simulink model "TDMA"  (R2021a)
settings: Solver=FixedStepDiscrete  StartTime=0.0  StopTime=1e-4  FixedStep=1/(sampling_freq*5)  RelTol=1e-3
undefined symbols (not defined in the file): coeff_t, data_rate, nco_2, nco_costasloopt, nco_t, sample_ratio, sampling_freq
libraries: simulink x64, simulink_extras x14, dspswit3 x14, commrandsrc3 x5
(part 1 of 2)
settings Model: Creator=Administrator  LastModifiedBy=Administrator

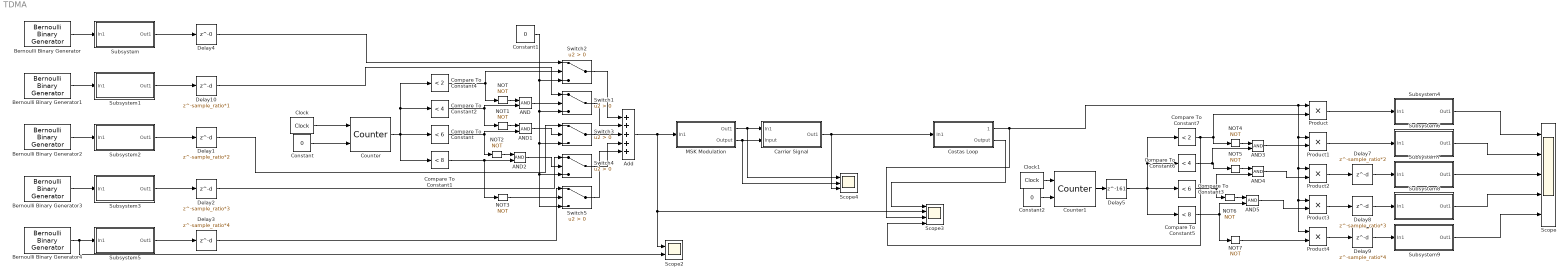
== system TDMA ==
  AND{,1..5} (6 alike) : Logic  IconShape=distinctive  AllPortsSameDT=off  OutDataTypeStr=boolean
  Add : Sum  Inputs=+++++
  Bernoulli Binary Generator{,1..4} (5 alike) : commrandsrc3/Bernoulli Binary Generator  ProbabilityOfZero=0.5  SeedSource=Parameter  Seed=23  SampleTime=1/data_rate  SamplesPerFrame=1  OutputDataType=boolean  SimulateUsing=Interpreted execution
  Carrier Signal : Subsystem
  Clock : simulink_extras/Flip Flops/Clock  period=10/sampling_freq
  Clock1 : simulink_extras/Flip Flops/Clock  period=10/sampling_freq
  Compare To Constant : simulink/Logic and Bit Operations/Compare To Constant  relop=<  const=6  OutDataTypeStr=boolean
  Compare To Constant1 : simulink/Logic and Bit Operations/Compare To Constant  relop=<  const=8  OutDataTypeStr=boolean
  Compare To Constant2 : simulink/Logic and Bit Operations/Compare To Constant  relop=<  const=4  OutDataTypeStr=boolean
  Compare To Constant3 : simulink/Logic and Bit Operations/Compare To Constant  relop=<  const=6  OutDataTypeStr=boolean
  Compare To Constant4 : simulink/Logic and Bit Operations/Compare To Constant  relop=<  const=2  OutDataTypeStr=boolean
  Compare To Constant5 : simulink/Logic and Bit Operations/Compare To Constant  relop=<  const=8  OutDataTypeStr=boolean
  Compare To Constant6 : simulink/Logic and Bit Operations/Compare To Constant  relop=<  const=4  OutDataTypeStr=boolean
  Compare To Constant7 : simulink/Logic and Bit Operations/Compare To Constant  relop=<  const=2  OutDataTypeStr=boolean
  Constant : Constant  Value=0
  Constant1 : Constant  Value=0  SampleTime=25e-9
  Constant2 : Constant  Value=0
  Costas Loop : Subsystem
  Counter : dspswit3/Counter  Direction=Up  CountEvent=Rising edge  CounterSize=User defined  MaxCount=9  InitialCount=0  Output=Count  HitValue=32  ResetInput=on  SamplesPerFrame=1  Ts=1  CntDtype=double  HitDtype=Logical
  Counter1 : dspswit3/Counter  Direction=Up  CountEvent=Rising edge  CounterSize=User defined  MaxCount=9  InitialCount=0  Output=Count  HitValue=32  ResetInput=on  SamplesPerFrame=1  Ts=1  CntDtype=double  HitDtype=Logical
  Delay1 : Delay  DelayLength=sample_ratio*2  SampleTime=1/sampling_freq
  Delay10 : Delay  DelayLength=sample_ratio*1  SampleTime=1/sampling_freq
  Delay2 : Delay  DelayLength=sample_ratio*3  SampleTime=1/sampling_freq
  Delay3 : Delay  DelayLength=sample_ratio*4  SampleTime=1/sampling_freq
  Delay4 : Delay  DelayLength=0  SampleTime=1/sampling_freq
  Delay5 : Delay  DelayLength=161  InitialCondition=0  UseCircularBuffer=on  SampleTime=1/(sampling_freq*5)
  Delay7 : Delay  DelayLength=sample_ratio*2  SampleTime=1/sampling_freq
  Delay8 : Delay  DelayLength=sample_ratio*3  SampleTime=1/sampling_freq
  Delay9 : Delay  DelayLength=sample_ratio*4  SampleTime=1/sampling_freq
  MSK Modulation : Subsystem
  NOT{,1..7} (8 alike) : Logic  Operator=NOT  IconShape=distinctive  AllPortsSameDT=off  OutDataTypeStr=boolean
  Product{,1..4} (5 alike) : Product
  Scope : Scope  NumInputPorts=5
  Scope2 : Scope  NumInputPorts=2
  Scope3 : Scope  NumInputPorts=4
  Scope4 : Scope  NumInputPorts=3
  Subsystem : Subsystem
  Subsystem1 : Subsystem
  Subsystem2 : Subsystem
  Subsystem3 : Subsystem
  Subsystem4 : Subsystem
  Subsystem5 : Subsystem
  Subsystem6 : Subsystem
  Subsystem7 : Subsystem
  Subsystem8 : Subsystem
  Subsystem9 : Subsystem
  Switch{1..5} (5 alike) : Switch  Criteria=u2 > Threshold  OutDataTypeStr=fixdt(1,32,29)  RndMeth=Nearest
  wires:
  Bernoulli Binary Generator/1 -> Subsystem/1(In1)
  Bernoulli Binary Generator1/1 -> Subsystem1/1(In1)
  Bernoulli Binary Generator2/1 -> Subsystem2/1(In1)
  Bernoulli Binary Generator3/1 -> Subsystem3/1(In1)
  Bernoulli Binary Generator4/1 -> Scope2/2, Subsystem5/1(In1)
  MSK Modulation/1(Out1) -> Scope4/1, Carrier Signal/1(In1)
  MSK Modulation/2(Output) -> Scope4/2, Carrier Signal/2(Input)
  Subsystem1/1(Out1) -> Delay10/1
  Subsystem2/1(Out1) -> Delay1/1
  Subsystem3/1(Out1) -> Delay2/1
  Subsystem5/1(Out1) -> Delay3/1
  Switch4/1 -> Add/4
  Switch1/1 -> Add/2
  Counter/1 -> Compare To Constant/1, Compare To Constant1/1, Compare To Constant4/1, Compare To Constant2/1
  Compare To Constant4/1 -> Switch2/2, NOT/1
  Constant1/1 -> Switch4/3, Switch5/3, Switch3/3, Switch1/3, Switch2/3
  Switch2/1 -> Add/1
  Switch3/1 -> Add/3
  Switch5/1 -> Add/5
  Subsystem/1(Out1) -> Delay4/1
  Clock/1 -> Counter/1
  AND/1 -> Switch1/2
  Compare To Constant2/1 -> NOT1/1, AND/2
  NOT/1 -> AND/1
  NOT1/1 -> AND1/1
  Compare To Constant/1 -> AND1/2, NOT2/1
  AND1/1 -> Switch3/2
  NOT2/1 -> AND2/1
  Compare To Constant1/1 -> NOT3/1, AND2/2
  AND2/1 -> Switch4/2
  Constant/1 -> Counter/2
  NOT3/1 -> Switch5/2
  Delay4/1 -> Switch2/1
  Delay10/1 -> Switch1/1
  Delay1/1 -> Switch3/1
  Delay2/1 -> Switch4/1
  Delay3/1 -> Switch5/1
  Constant2/1 -> Counter1/2
  Counter1/1 -> Delay5/1
  Clock1/1 -> Counter1/1
  NOT6/1 -> AND5/1
  NOT5/1 -> AND4/1
  NOT4/1 -> AND3/1
  Compare To Constant5/1 -> NOT7/1, AND5/2
  AND5/1 -> Product3/2
  NOT7/1 -> Product4/2
  Compare To Constant3/1 -> NOT6/1, AND4/2
  Compare To Constant6/1 -> AND3/2, NOT5/1
  Compare To Constant7/1 -> Scope3/4, NOT4/1, Product/2
  AND3/1 -> Product1/2
  AND4/1 -> Product2/2
  Add/1 -> Scope2/1, Scope3/2, MSK Modulation/1(In1)
  Carrier Signal/1(Out1) -> Scope4/3, Costas Loop/1(In1)
  Costas Loop/1(1) -> Scope3/3, Product2/1, Product3/1, Product4/1, Product1/1, Product/1
  Product/1 -> Subsystem4/1(In1)
  Costas Loop/2(Output) -> Scope3/1
  Delay5/1 -> Compare To Constant3/1, Compare To Constant5/1, Compare To Constant7/1, Compare To Constant6/1
  Product2/1 -> Delay7/1
  Product3/1 -> Delay8/1
  Product4/1 -> Delay9/1
  Product1/1 -> Subsystem6/1(In1)
  Delay7/1 -> Subsystem7/1(In1)
  Delay8/1 -> Subsystem8/1(In1)
  Delay9/1 -> Subsystem9/1(In1)
  Subsystem4/1(Out1) -> Scope/1
  Subsystem6/1(Out1) -> Scope/2
  Subsystem7/1(Out1) -> Scope/3
  Subsystem8/1(Out1) -> Scope/4
  Subsystem9/1(Out1) -> Scope/5

== system TDMA/Carrier Signal ==
  In1 : Inport
  Input : Inport  Port=2
  Add : Sum
  Data Type Conversion1 : DataTypeConversion  OutMin=[-1]  OutMax=[1]  OutDataTypeStr=fixdt(1,8)
  Data Type Conversion2 : DataTypeConversion  OutMin=[-1]  OutMax=[1]  OutDataTypeStr=fixdt(1,8)
  Data Type Conversion36 : DataTypeConversion  OutMin=[-2]  OutMax=[2]  OutDataTypeStr=fixdt(1,16)
  NCO : Subsystem
  Product2 : Product
  Product3 : Product
  Out1 : Outport
  wires:
  In1/1 -> Product3/2
  Data Type Conversion2/1 -> Product3/1
  NCO/1(Out2) -> Data Type Conversion2/1
  Product2/1 -> Add/2
  Add/1 -> Data Type Conversion36/1
  Product3/1 -> Add/1
  NCO/2(Out1) -> Data Type Conversion1/1
  Input/1 -> Product2/1
  Data Type Conversion1/1 -> Product2/2
  Data Type Conversion36/1 -> Out1/1

== system TDMA/Costas Loop ==
  In1 : Inport
  Compare To Constant4 : simulink/Logic and Bit Operations/Compare To Constant  relop=>  const=0  OutDataTypeStr=boolean
  Data Type Conversion{32..35,37..38} (6 alike) : DataTypeConversion  OutMin=[-2]  OutMax=[2]  OutDataTypeStr=fixdt(1,16)
  Filter1 : Subsystem  Tag=FilterWizardSubSystem
      settings: ErrorFcn=dspFilterRealizedInBasicElemsAlgLoopErrFcnCallback
  Filter2 : Subsystem  Tag=FilterWizardSubSystem
      settings: ErrorFcn=dspFilterRealizedInBasicElemsAlgLoopErrFcnCallback
  Filter3 : Subsystem  Tag=FilterWizardSubSystem
      settings: ErrorFcn=dspFilterRealizedInBasicElemsAlgLoopErrFcnCallback
  Gain : Gain  Gain=1/100
  NCO1 : Subsystem
  Product10 : Product
  Product11 : Product
  Product9 : Product
  Scope : Scope  NumInputPorts=2
  1 : Outport
  Output : Outport  Port=2
  wires:
  Data Type Conversion38/1 -> NCO1/1(In1)
  Data Type Conversion33/1 -> Product11/2
  Filter3/1(Output) -> Compare To Constant4/1, Product10/2, Output/1, Scope/1
  Filter1/1(Output) -> Product10/1, Scope/2
  Data Type Conversion32/1 -> Filter3/1(Input)
  Data Type Conversion34/1 -> Product9/1
  Filter2/1(Output) -> Gain/1
  NCO1/1(Out1) -> Product9/2
  Data Type Conversion37/1 -> Filter2/1(Input)
  In1/1 -> Data Type Conversion34/1, Data Type Conversion33/1
  Gain/1 -> Data Type Conversion38/1
  Product10/1 -> Data Type Conversion37/1
  Product11/1 -> Data Type Conversion32/1
  Data Type Conversion35/1 -> Filter1/1(Input)
  Compare To Constant4/1 -> 1/1
  Product9/1 -> Data Type Conversion35/1
  NCO1/2(sin(2*pi*u)) -> Product11/1

== system TDMA/MSK Modulation ==
  In1 : Inport
  Add1 : Sum
  Add2 : Sum
  Constant : Constant  Value=-1
  Constant1 : Constant  Value=2
  Constant2 : Constant  Value=-1
  Constant3 : Constant  Value=2
  Data Type Conversion : DataTypeConversion  OutDataTypeStr=boolean
  Data Type Conversion{3..6} (4 alike) : DataTypeConversion  OutMin=[-1]  OutMax=[1]  OutDataTypeStr=fixdt(1,8)
  Delay : Delay  DelayLength=sample_ratio  SampleTime=1/(sampling_freq*5)
  Delay1 : Delay  DelayLength=sample_ratio  SampleTime=1/(sampling_freq*5)
  NCO2 : Subsystem
  Product{,1,4..5} (4 alike) : Product
  clock : DiscretePulseGenerator  PulseType=Time based  Period=2/(sampling_freq*5)  PulseWidth=50
  rate transition1 : Subsystem
  rate transition3 : Subsystem
  Out1 : Outport
  Output : Outport  Port=2
  wires:
  NCO2/2(Out1) -> Data Type Conversion3/1
  Delay/1 -> rate transition1/1(In1)
  Delay1/1 -> Product4/2
  rate transition1/1(Out1) -> Product5/2
  rate transition3/1(Out1) -> Delay1/1
  NCO2/1(Out2) -> Data Type Conversion6/1
  Data Type Conversion6/1 -> Product1/1
  Add2/1 -> Data Type Conversion4/1
  Data Type Conversion4/1 -> Product/1
  Data Type Conversion3/1 -> Product/2
  Constant1/1 -> Product4/1
  Data Type Conversion5/1 -> Product1/2
  Add1/1 -> Data Type Conversion5/1
  Product5/1 -> Add2/2
  Data Type Conversion/1 -> rate transition3/1(In1), Delay/1
  clock/1 -> rate transition1/2(In2), rate transition3/2(In2)
  Constant2/1 -> Add2/1
  Constant/1 -> Add1/1
  Constant3/1 -> Product5/1
  Product4/1 -> Add1/2
  Product1/1 -> Out1/1
  Product/1 -> Output/1
  In1/1 -> Data Type Conversion/1

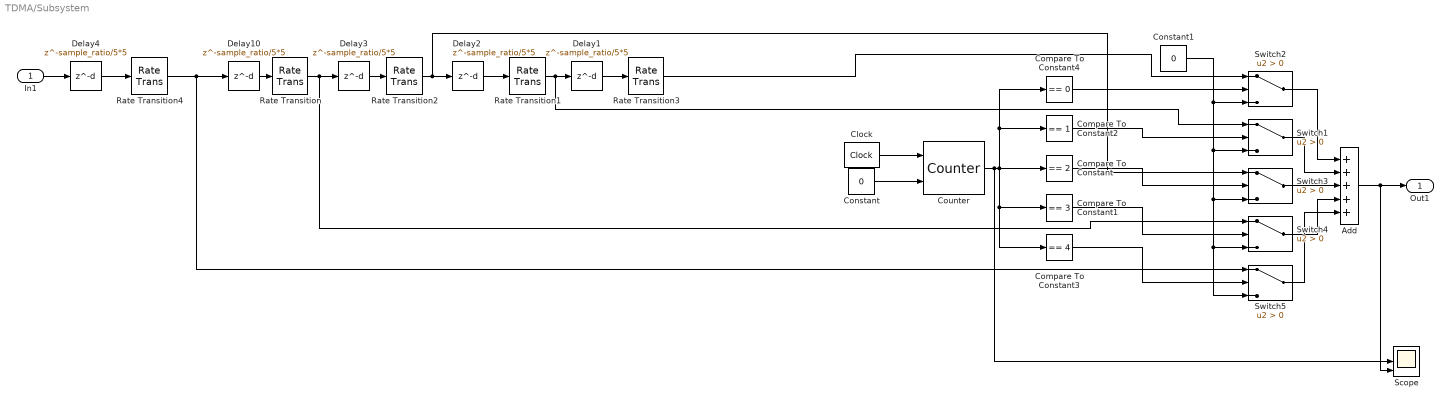
== system TDMA/Subsystem ==
  In1 : Inport
  Add : Sum  Inputs=+++++
  Clock : simulink_extras/Flip Flops/Clock  period=4/sampling_freq
  Compare To Constant : simulink/Logic and Bit Operations/Compare To Constant  relop===  const=2  OutDataTypeStr=boolean
  Compare To Constant1 : simulink/Logic and Bit Operations/Compare To Constant  relop===  const=3  OutDataTypeStr=boolean
  Compare To Constant2 : simulink/Logic and Bit Operations/Compare To Constant  relop===  const=1  OutDataTypeStr=boolean
  Compare To Constant3 : simulink/Logic and Bit Operations/Compare To Constant  relop===  const=4  OutDataTypeStr=boolean
  Compare To Constant4 : simulink/Logic and Bit Operations/Compare To Constant  relop===  const=0  OutDataTypeStr=boolean
  Constant : Constant  Value=0
  Constant1 : Constant  Value=0  SampleTime=25e-9
  Counter : dspswit3/Counter  Direction=Up  CountEvent=Rising edge  CounterSize=User defined  MaxCount=4  InitialCount=0  Output=Count  HitValue=32  ResetInput=on  SamplesPerFrame=1  Ts=1  CntDtype=double  HitDtype=Logical
  Delay{1..4,10} (5 alike) : Delay  DelayLength=sample_ratio/5*5  SampleTime=1/sampling_freq
  Rate Transition{,1..4} (5 alike) : RateTransition  OutPortSampleTime=1/data_rate
  Scope : Scope  NumInputPorts=3
  Switch{1..5} (5 alike) : Switch  Criteria=u2 > Threshold  OutDataTypeStr=fixdt(1,32,29)  RndMeth=Nearest
  Out1 : Outport
  wires:
  Rate Transition1/1 -> Switch1/1, Delay1/1
  Switch2/1 -> Add/1
  Counter/1 -> Scope/2, Compare To Constant/1, Compare To Constant3/1, Compare To Constant1/1, Compare To Constant4/1, Compare To Constant2/1
  Delay2/1 -> Rate Transition1/1
  Add/1 -> Scope/3, Out1/1
  Constant/1 -> Counter/2
  Switch3/1 -> Add/3
  Constant1/1 -> Switch4/3, Switch5/3, Switch3/3, Switch1/3, Switch2/3
  Switch5/1 -> Add/5
  Rate Transition/1 -> Switch4/1, Delay3/1
  Switch4/1 -> Add/4
  Delay3/1 -> Rate Transition2/1
  Compare To Constant2/1 -> Switch1/2
  Compare To Constant3/1 -> Switch5/2
  Compare To Constant/1 -> Switch3/2
  Switch1/1 -> Add/2
  Clock/1 -> Counter/1
  Compare To Constant1/1 -> Switch4/2
  Delay1/1 -> Rate Transition3/1
  Rate Transition2/1 -> Switch3/1, Delay2/1
  Compare To Constant4/1 -> Switch2/2
  Delay10/1 -> Rate Transition/1
  In1/1 -> Delay4/1
  Rate Transition3/1 -> Switch2/1
  Rate Transition4/1 -> Switch5/1, Delay10/1
  Delay4/1 -> Rate Transition4/1

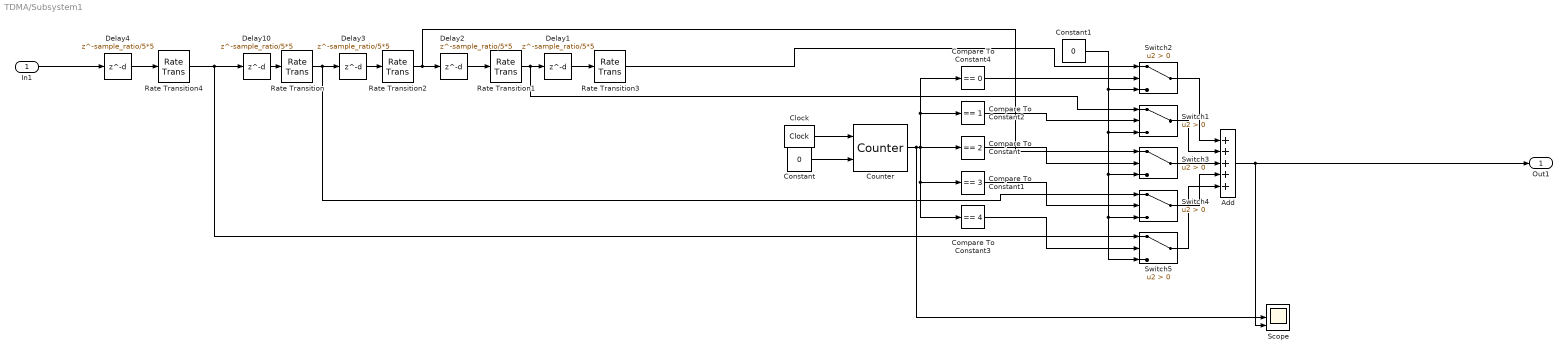
== system TDMA/Subsystem1 ==
  In1 : Inport
  Add : Sum  Inputs=+++++
  Clock : simulink_extras/Flip Flops/Clock  period=4/sampling_freq
  Compare To Constant : simulink/Logic and Bit Operations/Compare To Constant  relop===  const=2  OutDataTypeStr=boolean
  Compare To Constant1 : simulink/Logic and Bit Operations/Compare To Constant  relop===  const=3  OutDataTypeStr=boolean
  Compare To Constant2 : simulink/Logic and Bit Operations/Compare To Constant  relop===  const=1  OutDataTypeStr=boolean
  Compare To Constant3 : simulink/Logic and Bit Operations/Compare To Constant  relop===  const=4  OutDataTypeStr=boolean
  Compare To Constant4 : simulink/Logic and Bit Operations/Compare To Constant  relop===  const=0  OutDataTypeStr=boolean
  Constant : Constant  Value=0
  Constant1 : Constant  Value=0  SampleTime=25e-9
  Counter : dspswit3/Counter  Direction=Up  CountEvent=Rising edge  CounterSize=User defined  MaxCount=4  InitialCount=0  Output=Count  HitValue=32  ResetInput=on  SamplesPerFrame=1  Ts=1  CntDtype=double  HitDtype=Logical
  Delay{1..4,10} (5 alike) : Delay  DelayLength=sample_ratio/5*5  SampleTime=1/sampling_freq
  Rate Transition{,1..4} (5 alike) : RateTransition  OutPortSampleTime=1/data_rate
  Scope : Scope  NumInputPorts=3
  Switch{1..5} (5 alike) : Switch  Criteria=u2 > Threshold  OutDataTypeStr=fixdt(1,32,29)  RndMeth=Nearest
  Out1 : Outport
  wires:
  Rate Transition1/1 -> Switch1/1, Delay1/1
  Switch2/1 -> Add/1
  Counter/1 -> Scope/2, Compare To Constant/1, Compare To Constant3/1, Compare To Constant1/1, Compare To Constant4/1, Compare To Constant2/1
  Delay2/1 -> Rate Transition1/1
  Add/1 -> Scope/3, Out1/1
  Constant/1 -> Counter/2
  Switch3/1 -> Add/3
  Constant1/1 -> Switch4/3, Switch5/3, Switch3/3, Switch1/3, Switch2/3
  Switch5/1 -> Add/5
  Rate Transition/1 -> Switch4/1, Delay3/1
  Switch4/1 -> Add/4
  Delay3/1 -> Rate Transition2/1
  Compare To Constant2/1 -> Switch1/2
  Compare To Constant3/1 -> Switch5/2
  Compare To Constant/1 -> Switch3/2
  Switch1/1 -> Add/2
  Clock/1 -> Counter/1
  Compare To Constant1/1 -> Switch4/2
  Delay1/1 -> Rate Transition3/1
  Rate Transition2/1 -> Switch3/1, Delay2/1
  Compare To Constant4/1 -> Switch2/2
  Delay10/1 -> Rate Transition/1
  In1/1 -> Delay4/1
  Rate Transition3/1 -> Switch2/1
  Rate Transition4/1 -> Switch5/1, Delay10/1
  Delay4/1 -> Rate Transition4/1

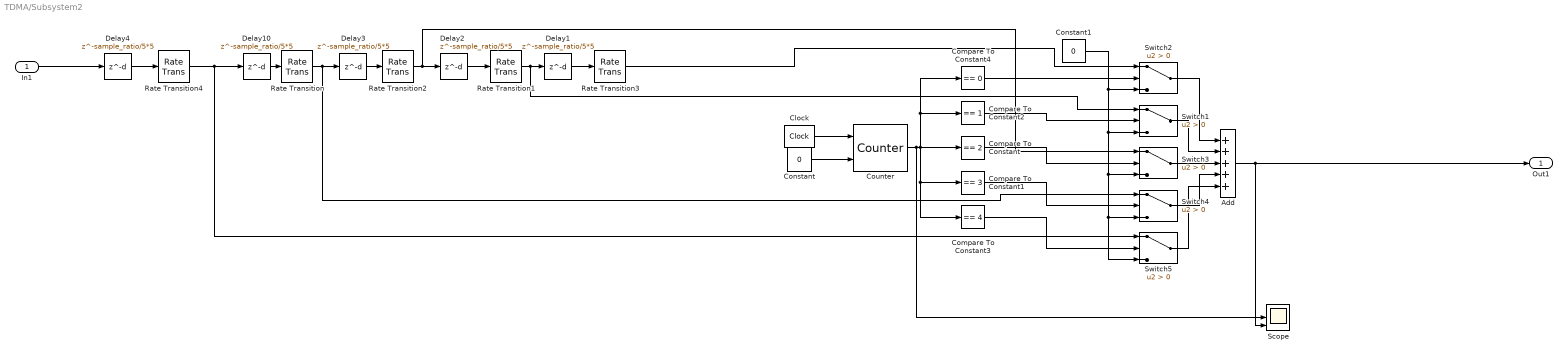
== system TDMA/Subsystem2 ==
  In1 : Inport
  Add : Sum  Inputs=+++++
  Clock : simulink_extras/Flip Flops/Clock  period=4/sampling_freq
  Compare To Constant : simulink/Logic and Bit Operations/Compare To Constant  relop===  const=2  OutDataTypeStr=boolean
  Compare To Constant1 : simulink/Logic and Bit Operations/Compare To Constant  relop===  const=3  OutDataTypeStr=boolean
  Compare To Constant2 : simulink/Logic and Bit Operations/Compare To Constant  relop===  const=1  OutDataTypeStr=boolean
  Compare To Constant3 : simulink/Logic and Bit Operations/Compare To Constant  relop===  const=4  OutDataTypeStr=boolean
  Compare To Constant4 : simulink/Logic and Bit Operations/Compare To Constant  relop===  const=0  OutDataTypeStr=boolean
  Constant : Constant  Value=0
  Constant1 : Constant  Value=0  SampleTime=25e-9
  Counter : dspswit3/Counter  Direction=Up  CountEvent=Rising edge  CounterSize=User defined  MaxCount=4  InitialCount=0  Output=Count  HitValue=32  ResetInput=on  SamplesPerFrame=1  Ts=1  CntDtype=double  HitDtype=Logical
  Delay{1..4,10} (5 alike) : Delay  DelayLength=sample_ratio/5*5  SampleTime=1/sampling_freq
  Rate Transition{,1..4} (5 alike) : RateTransition  OutPortSampleTime=1/data_rate
  Scope : Scope  NumInputPorts=3
  Switch{1..5} (5 alike) : Switch  Criteria=u2 > Threshold  OutDataTypeStr=fixdt(1,32,29)  RndMeth=Nearest
  Out1 : Outport
  wires:
  Rate Transition1/1 -> Switch1/1, Delay1/1
  Switch2/1 -> Add/1
  Counter/1 -> Scope/2, Compare To Constant/1, Compare To Constant3/1, Compare To Constant1/1, Compare To Constant4/1, Compare To Constant2/1
  Delay2/1 -> Rate Transition1/1
  Add/1 -> Scope/3, Out1/1
  Constant/1 -> Counter/2
  Switch3/1 -> Add/3
  Constant1/1 -> Switch4/3, Switch5/3, Switch3/3, Switch1/3, Switch2/3
  Switch5/1 -> Add/5
  Rate Transition/1 -> Switch4/1, Delay3/1
  Switch4/1 -> Add/4
  Delay3/1 -> Rate Transition2/1
  Compare To Constant2/1 -> Switch1/2
  Compare To Constant3/1 -> Switch5/2
  Compare To Constant/1 -> Switch3/2
  Switch1/1 -> Add/2
  Clock/1 -> Counter/1
  Compare To Constant1/1 -> Switch4/2
  Delay1/1 -> Rate Transition3/1
  Rate Transition2/1 -> Switch3/1, Delay2/1
  Compare To Constant4/1 -> Switch2/2
  Delay10/1 -> Rate Transition/1
  In1/1 -> Delay4/1
  Rate Transition3/1 -> Switch2/1
  Rate Transition4/1 -> Switch5/1, Delay10/1
  Delay4/1 -> Rate Transition4/1

== system TDMA/Subsystem3 ==
  In1 : Inport
  Add : Sum  Inputs=+++++
  Clock : simulink_extras/Flip Flops/Clock  period=4/sampling_freq
  Compare To Constant : simulink/Logic and Bit Operations/Compare To Constant  relop===  const=2  OutDataTypeStr=boolean
  Compare To Constant1 : simulink/Logic and Bit Operations/Compare To Constant  relop===  const=3  OutDataTypeStr=boolean
  Compare To Constant2 : simulink/Logic and Bit Operations/Compare To Constant  relop===  const=1  OutDataTypeStr=boolean
  Compare To Constant3 : simulink/Logic and Bit Operations/Compare To Constant  relop===  const=4  OutDataTypeStr=boolean
  Compare To Constant4 : simulink/Logic and Bit Operations/Compare To Constant  relop===  const=0  OutDataTypeStr=boolean
  Constant : Constant  Value=0
  Constant1 : Constant  Value=0  SampleTime=25e-9
  Counter : dspswit3/Counter  Direction=Up  CountEvent=Rising edge  CounterSize=User defined  MaxCount=4  InitialCount=0  Output=Count  HitValue=32  ResetInput=on  SamplesPerFrame=1  Ts=1  CntDtype=double  HitDtype=Logical
  Delay{1..4,10} (5 alike) : Delay  DelayLength=sample_ratio/5*5  SampleTime=1/sampling_freq
  Rate Transition{,1..4} (5 alike) : RateTransition  OutPortSampleTime=1/data_rate
  Scope : Scope  NumInputPorts=3
  Switch{1..5} (5 alike) : Switch  Criteria=u2 > Threshold  OutDataTypeStr=fixdt(1,32,29)  RndMeth=Nearest
  Out1 : Outport
  wires:
  Rate Transition1/1 -> Switch1/1, Delay1/1
  Switch2/1 -> Add/1
  Counter/1 -> Scope/2, Compare To Constant/1, Compare To Constant3/1, Compare To Constant1/1, Compare To Constant4/1, Compare To Constant2/1
  Delay2/1 -> Rate Transition1/1
  Add/1 -> Scope/3, Out1/1
  Constant/1 -> Counter/2
  Switch3/1 -> Add/3
  Constant1/1 -> Switch4/3, Switch5/3, Switch3/3, Switch1/3, Switch2/3
  Switch5/1 -> Add/5
  Rate Transition/1 -> Switch4/1, Delay3/1
  Switch4/1 -> Add/4
  Delay3/1 -> Rate Transition2/1
  Compare To Constant2/1 -> Switch1/2
  Compare To Constant3/1 -> Switch5/2
  Compare To Constant/1 -> Switch3/2
  Switch1/1 -> Add/2
  Clock/1 -> Counter/1
  Compare To Constant1/1 -> Switch4/2
  Delay1/1 -> Rate Transition3/1
  Rate Transition2/1 -> Switch3/1, Delay2/1
  Compare To Constant4/1 -> Switch2/2
  Delay10/1 -> Rate Transition/1
  In1/1 -> Delay4/1
  Rate Transition3/1 -> Switch2/1
  Rate Transition4/1 -> Switch5/1, Delay10/1
  Delay4/1 -> Rate Transition4/1

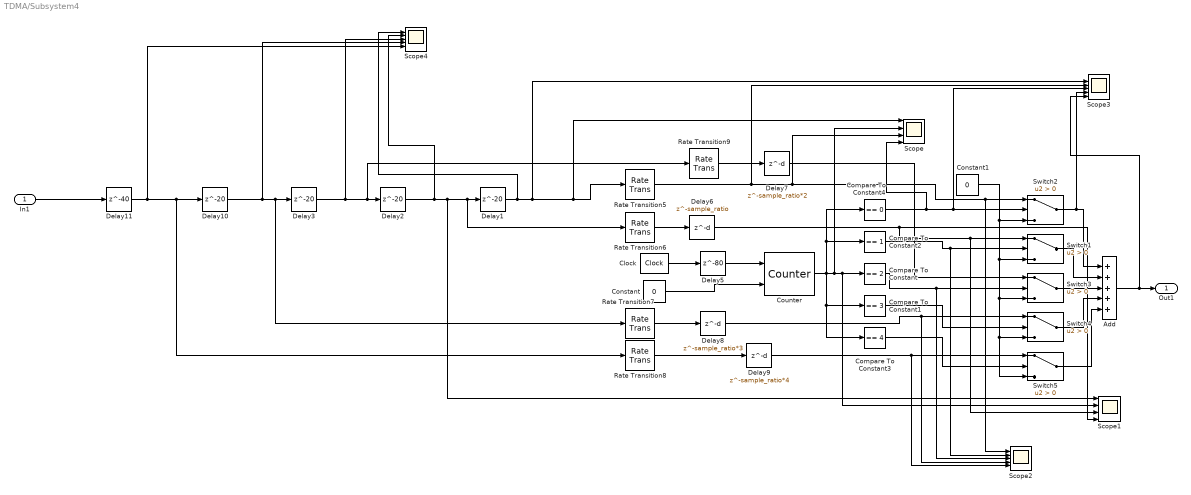
== system TDMA/Subsystem4 ==
  In1 : Inport
  Add : Sum  Inputs=+++++
  Clock : simulink_extras/Flip Flops/Clock  period=5*4/(sampling_freq)
  Compare To Constant : simulink/Logic and Bit Operations/Compare To Constant  relop===  const=2  OutDataTypeStr=boolean
  Compare To Constant1 : simulink/Logic and Bit Operations/Compare To Constant  relop===  const=3  OutDataTypeStr=boolean
  Compare To Constant2 : simulink/Logic and Bit Operations/Compare To Constant  relop===  const=1  OutDataTypeStr=boolean
  Compare To Constant3 : simulink/Logic and Bit Operations/Compare To Constant  relop===  const=4  OutDataTypeStr=boolean
  Compare To Constant4 : simulink/Logic and Bit Operations/Compare To Constant  relop===  const=0  OutDataTypeStr=boolean
  Constant : Constant  Value=0
  Constant1 : Constant  Value=0  SampleTime=25e-9
  Counter : dspswit3/Counter  Direction=Up  CountEvent=Rising edge  CounterSize=User defined  MaxCount=4  InitialCount=0  Output=Count  HitValue=32  ResetInput=on  SamplesPerFrame=1  Ts=1  CntDtype=double  HitDtype=Logical
  Delay{1..3,10} (4 alike) : Delay  DelayLength=20  SampleTime=1/(sampling_freq*5)
  Delay11 : Delay  DelayLength=40  SampleTime=1/(sampling_freq*5)
  Delay5 : Delay  DelayLength=80  SampleTime=1/(sampling_freq)
  Delay6 : Delay  DelayLength=sample_ratio  SampleTime=1/(sampling_freq)
  Delay7 : Delay  DelayLength=sample_ratio*2  SampleTime=1/(sampling_freq)
  Delay8 : Delay  DelayLength=sample_ratio*3  SampleTime=1/(sampling_freq)
  Delay9 : Delay  DelayLength=sample_ratio*4  SampleTime=1/(sampling_freq)
  Rate Transition{5..9} (5 alike) : RateTransition  OutPortSampleTime=1/(data_rate)
  Scope : Scope  NumInputPorts=4
  Scope1 : Scope  NumInputPorts=4
  Scope2 : Scope  NumInputPorts=5
  Scope3 : Scope  NumInputPorts=6
  Scope4 : Scope  NumInputPorts=5
  Switch{1..5} (5 alike) : Switch  Criteria=u2 > Threshold  OutDataTypeStr=fixdt(1,32,29)  RndMeth=Nearest
  Out1 : Outport
  wires:
  Switch2/1 -> Scope3/5, Add/1
  Counter/1 -> Scope/2, Scope1/2, Compare To Constant/1, Compare To Constant3/1, Compare To Constant1/1, Compare To Constant4/1, Compare To Constant2/1
  Add/1 -> Scope3/6, Out1/1
  Constant/1 -> Counter/2
  Switch3/1 -> Add/3
  Constant1/1 -> Switch4/3, Switch5/3, Switch3/3, Switch1/3, Switch2/3
  Switch5/1 -> Add/5
  Switch4/1 -> Add/4
  Compare To Constant2/1 -> Scope2/2, Switch1/2
  Compare To Constant3/1 -> Switch5/2
  Compare To Constant/1 -> Scope2/3, Switch3/2
  Switch1/1 -> Add/2
  Compare To Constant1/1 -> Switch4/2
  Compare To Constant4/1 -> Scope/4, Scope3/4, Switch2/2
  Delay1/1 -> Scope4/1, Scope3/2, Scope/1, Rate Transition5/1
  Rate Transition6/1 -> Delay6/1
  Rate Transition7/1 -> Delay8/1
  Rate Transition8/1 -> Delay9/1
  Rate Transition9/1 -> Delay7/1
  Clock/1 -> Delay5/1
  Delay5/1 -> Counter/1
  Delay2/1 -> Scope4/2, Scope1/1, Rate Transition6/1, Delay1/1
  Delay3/1 -> Scope4/3, Rate Transition9/1, Delay2/1
  Delay10/1 -> Scope4/4, Rate Transition7/1, Delay3/1
  Delay6/1 -> Scope1/4, Scope1/3, Switch1/1
  Delay7/1 -> Switch3/1
  Delay8/1 -> Scope2/4, Switch4/1
  Delay9/1 -> Scope2/5, Switch5/1
  Rate Transition5/1 -> Scope3/3, Scope2/1, Switch2/1, Scope/3
  In1/1 -> Delay11/1
  Delay11/1 -> Scope4/5, Rate Transition8/1, Delay10/1

== system TDMA/Subsystem5 ==
  In1 : Inport
  Add : Sum  Inputs=+++++
  Clock : simulink_extras/Flip Flops/Clock  period=4/sampling_freq
  Compare To Constant : simulink/Logic and Bit Operations/Compare To Constant  relop===  const=2  OutDataTypeStr=boolean
  Compare To Constant1 : simulink/Logic and Bit Operations/Compare To Constant  relop===  const=3  OutDataTypeStr=boolean
  Compare To Constant2 : simulink/Logic and Bit Operations/Compare To Constant  relop===  const=1  OutDataTypeStr=boolean
  Compare To Constant3 : simulink/Logic and Bit Operations/Compare To Constant  relop===  const=4  OutDataTypeStr=boolean
  Compare To Constant4 : simulink/Logic and Bit Operations/Compare To Constant  relop===  const=0  OutDataTypeStr=boolean
  Constant : Constant  Value=0
  Constant1 : Constant  Value=0  SampleTime=25e-9
  Counter : dspswit3/Counter  Direction=Up  CountEvent=Rising edge  CounterSize=User defined  MaxCount=4  InitialCount=0  Output=Count  HitValue=32  ResetInput=on  SamplesPerFrame=1  Ts=1  CntDtype=double  HitDtype=Logical
  Delay{1..4,10} (5 alike) : Delay  DelayLength=sample_ratio/5*5  SampleTime=1/sampling_freq
  Rate Transition{,1..4} (5 alike) : RateTransition  OutPortSampleTime=1/data_rate
  Scope : Scope  NumInputPorts=3
  Switch{1..5} (5 alike) : Switch  Criteria=u2 > Threshold  OutDataTypeStr=fixdt(1,32,29)  RndMeth=Nearest
  Out1 : Outport
  wires:
  Rate Transition1/1 -> Switch1/1, Delay1/1
  Switch2/1 -> Add/1
  Counter/1 -> Scope/2, Compare To Constant/1, Compare To Constant3/1, Compare To Constant1/1, Compare To Constant4/1, Compare To Constant2/1
  Delay2/1 -> Rate Transition1/1
  Add/1 -> Scope/3, Out1/1
  Constant/1 -> Counter/2
  Switch3/1 -> Add/3
  Constant1/1 -> Switch4/3, Switch5/3, Switch3/3, Switch1/3, Switch2/3
  Switch5/1 -> Add/5
  Rate Transition/1 -> Switch4/1, Delay3/1
  Switch4/1 -> Add/4
  Delay3/1 -> Rate Transition2/1
  Compare To Constant2/1 -> Switch1/2
  Compare To Constant3/1 -> Switch5/2
  Compare To Constant/1 -> Switch3/2
  Switch1/1 -> Add/2
  Clock/1 -> Counter/1
  Compare To Constant1/1 -> Switch4/2
  Delay1/1 -> Rate Transition3/1
  Rate Transition2/1 -> Switch3/1, Delay2/1
  Compare To Constant4/1 -> Switch2/2
  Delay10/1 -> Rate Transition/1
  In1/1 -> Delay4/1
  Rate Transition3/1 -> Switch2/1
  Rate Transition4/1 -> Switch5/1, Delay10/1
  Delay4/1 -> Rate Transition4/1

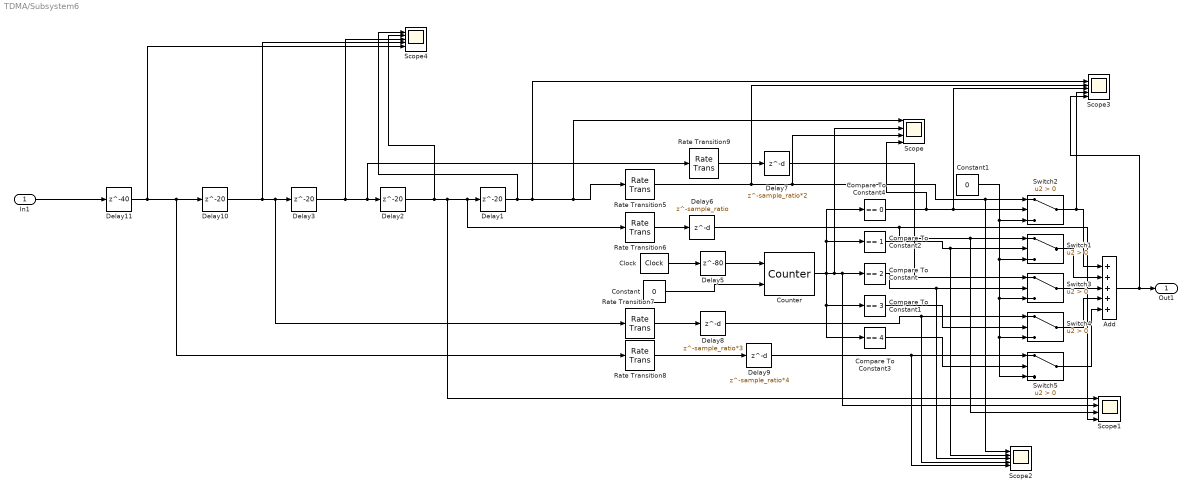
== system TDMA/Subsystem6 ==
  In1 : Inport
  Add : Sum  Inputs=+++++
  Clock : simulink_extras/Flip Flops/Clock  period=5*4/(sampling_freq)
  Compare To Constant : simulink/Logic and Bit Operations/Compare To Constant  relop===  const=2  OutDataTypeStr=boolean
  Compare To Constant1 : simulink/Logic and Bit Operations/Compare To Constant  relop===  const=3  OutDataTypeStr=boolean
  Compare To Constant2 : simulink/Logic and Bit Operations/Compare To Constant  relop===  const=1  OutDataTypeStr=boolean
  Compare To Constant3 : simulink/Logic and Bit Operations/Compare To Constant  relop===  const=4  OutDataTypeStr=boolean
  Compare To Constant4 : simulink/Logic and Bit Operations/Compare To Constant  relop===  const=0  OutDataTypeStr=boolean
  Constant : Constant  Value=0
  Constant1 : Constant  Value=0  SampleTime=25e-9
  Counter : dspswit3/Counter  Direction=Up  CountEvent=Rising edge  CounterSize=User defined  MaxCount=4  InitialCount=0  Output=Count  HitValue=32  ResetInput=on  SamplesPerFrame=1  Ts=1  CntDtype=double  HitDtype=Logical
  Delay{1..3,10} (4 alike) : Delay  DelayLength=20  SampleTime=1/(sampling_freq*5)
  Delay11 : Delay  DelayLength=40  SampleTime=1/(sampling_freq*5)
  Delay5 : Delay  DelayLength=80  SampleTime=1/(sampling_freq)
  Delay6 : Delay  DelayLength=sample_ratio  SampleTime=1/(sampling_freq)
  Delay7 : Delay  DelayLength=sample_ratio*2  SampleTime=1/(sampling_freq)
  Delay8 : Delay  DelayLength=sample_ratio*3  SampleTime=1/(sampling_freq)
  Delay9 : Delay  DelayLength=sample_ratio*4  SampleTime=1/(sampling_freq)
  Rate Transition{5..9} (5 alike) : RateTransition  OutPortSampleTime=1/(data_rate)
  Scope : Scope  NumInputPorts=4
  Scope1 : Scope  NumInputPorts=4
  Scope2 : Scope  NumInputPorts=5
  Scope3 : Scope  NumInputPorts=6
  Scope4 : Scope  NumInputPorts=5
  Switch{1..5} (5 alike) : Switch  Criteria=u2 > Threshold  OutDataTypeStr=fixdt(1,32,29)  RndMeth=Nearest
  Out1 : Outport
  wires:
  Switch2/1 -> Scope3/5, Add/1
  Counter/1 -> Scope/2, Scope1/2, Compare To Constant/1, Compare To Constant3/1, Compare To Constant1/1, Compare To Constant4/1, Compare To Constant2/1
  Add/1 -> Scope3/6, Out1/1
  Constant/1 -> Counter/2
  Switch3/1 -> Add/3
  Constant1/1 -> Switch4/3, Switch5/3, Switch3/3, Switch1/3, Switch2/3
  Switch5/1 -> Add/5
  Switch4/1 -> Add/4
  Compare To Constant2/1 -> Scope2/2, Switch1/2
  Compare To Constant3/1 -> Switch5/2
  Compare To Constant/1 -> Scope2/3, Switch3/2
  Switch1/1 -> Add/2
  Compare To Constant1/1 -> Switch4/2
  Compare To Constant4/1 -> Scope/4, Scope3/4, Switch2/2
  Delay1/1 -> Scope4/1, Scope3/2, Scope/1, Rate Transition5/1
  Rate Transition6/1 -> Delay6/1
  Rate Transition7/1 -> Delay8/1
  Rate Transition8/1 -> Delay9/1
  Rate Transition9/1 -> Delay7/1
  Clock/1 -> Delay5/1
  Delay5/1 -> Counter/1
  Delay2/1 -> Scope4/2, Scope1/1, Rate Transition6/1, Delay1/1
  Delay3/1 -> Scope4/3, Rate Transition9/1, Delay2/1
  Delay10/1 -> Scope4/4, Rate Transition7/1, Delay3/1
  Delay6/1 -> Scope1/4, Scope1/3, Switch1/1
  Delay7/1 -> Switch3/1
  Delay8/1 -> Scope2/4, Switch4/1
  Delay9/1 -> Scope2/5, Switch5/1
  Rate Transition5/1 -> Scope3/3, Scope2/1, Switch2/1, Scope/3
  In1/1 -> Delay11/1
  Delay11/1 -> Scope4/5, Rate Transition8/1, Delay10/1

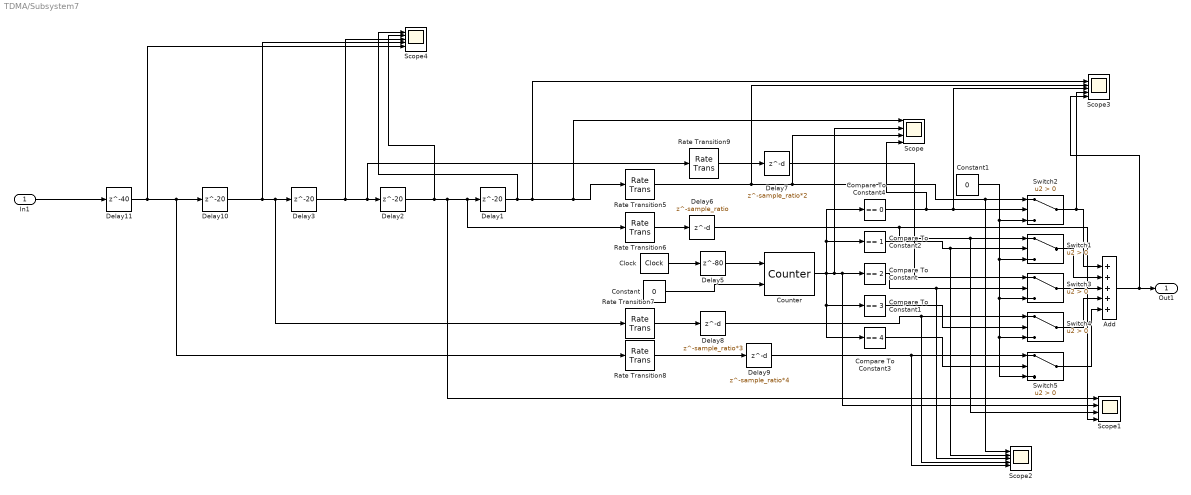
== system TDMA/Subsystem7 ==
  In1 : Inport
  Add : Sum  Inputs=+++++
  Clock : simulink_extras/Flip Flops/Clock  period=5*4/(sampling_freq)
  Compare To Constant : simulink/Logic and Bit Operations/Compare To Constant  relop===  const=2  OutDataTypeStr=boolean
  Compare To Constant1 : simulink/Logic and Bit Operations/Compare To Constant  relop===  const=3  OutDataTypeStr=boolean
  Compare To Constant2 : simulink/Logic and Bit Operations/Compare To Constant  relop===  const=1  OutDataTypeStr=boolean
  Compare To Constant3 : simulink/Logic and Bit Operations/Compare To Constant  relop===  const=4  OutDataTypeStr=boolean
  Compare To Constant4 : simulink/Logic and Bit Operations/Compare To Constant  relop===  const=0  OutDataTypeStr=boolean
  Constant : Constant  Value=0
  Constant1 : Constant  Value=0  SampleTime=25e-9
  Counter : dspswit3/Counter  Direction=Up  CountEvent=Rising edge  CounterSize=User defined  MaxCount=4  InitialCount=0  Output=Count  HitValue=32  ResetInput=on  SamplesPerFrame=1  Ts=1  CntDtype=double  HitDtype=Logical
  Delay{1..3,10} (4 alike) : Delay  DelayLength=20  SampleTime=1/(sampling_freq*5)
  Delay11 : Delay  DelayLength=40  SampleTime=1/(sampling_freq*5)
  Delay5 : Delay  DelayLength=80  SampleTime=1/(sampling_freq)
  Delay6 : Delay  DelayLength=sample_ratio  SampleTime=1/(sampling_freq)
  Delay7 : Delay  DelayLength=sample_ratio*2  SampleTime=1/(sampling_freq)
  Delay8 : Delay  DelayLength=sample_ratio*3  SampleTime=1/(sampling_freq)
  Delay9 : Delay  DelayLength=sample_ratio*4  SampleTime=1/(sampling_freq)
  Rate Transition{5..9} (5 alike) : RateTransition  OutPortSampleTime=1/(data_rate)
  Scope : Scope  NumInputPorts=4
  Scope1 : Scope  NumInputPorts=4
  Scope2 : Scope  NumInputPorts=5
  Scope3 : Scope  NumInputPorts=6
  Scope4 : Scope  NumInputPorts=5
  Switch{1..5} (5 alike) : Switch  Criteria=u2 > Threshold  OutDataTypeStr=fixdt(1,32,29)  RndMeth=Nearest
  Out1 : Outport
  wires:
  Switch2/1 -> Scope3/5, Add/1
  Counter/1 -> Scope/2, Scope1/2, Compare To Constant/1, Compare To Constant3/1, Compare To Constant1/1, Compare To Constant4/1, Compare To Constant2/1
  Add/1 -> Scope3/6, Out1/1
  Constant/1 -> Counter/2
  Switch3/1 -> Add/3
  Constant1/1 -> Switch4/3, Switch5/3, Switch3/3, Switch1/3, Switch2/3
  Switch5/1 -> Add/5
  Switch4/1 -> Add/4
  Compare To Constant2/1 -> Scope2/2, Switch1/2
  Compare To Constant3/1 -> Switch5/2
  Compare To Constant/1 -> Scope2/3, Switch3/2
  Switch1/1 -> Add/2
  Compare To Constant1/1 -> Switch4/2
  Compare To Constant4/1 -> Scope/4, Scope3/4, Switch2/2
  Delay1/1 -> Scope4/1, Scope3/2, Scope/1, Rate Transition5/1
  Rate Transition6/1 -> Delay6/1
  Rate Transition7/1 -> Delay8/1
  Rate Transition8/1 -> Delay9/1
  Rate Transition9/1 -> Delay7/1
  Clock/1 -> Delay5/1
  Delay5/1 -> Counter/1
  Delay2/1 -> Scope4/2, Scope1/1, Rate Transition6/1, Delay1/1
  Delay3/1 -> Scope4/3, Rate Transition9/1, Delay2/1
  Delay10/1 -> Scope4/4, Rate Transition7/1, Delay3/1
  Delay6/1 -> Scope1/4, Scope1/3, Switch1/1
  Delay7/1 -> Switch3/1
  Delay8/1 -> Scope2/4, Switch4/1
  Delay9/1 -> Scope2/5, Switch5/1
  Rate Transition5/1 -> Scope3/3, Scope2/1, Switch2/1, Scope/3
  In1/1 -> Delay11/1
  Delay11/1 -> Scope4/5, Rate Transition8/1, Delay10/1

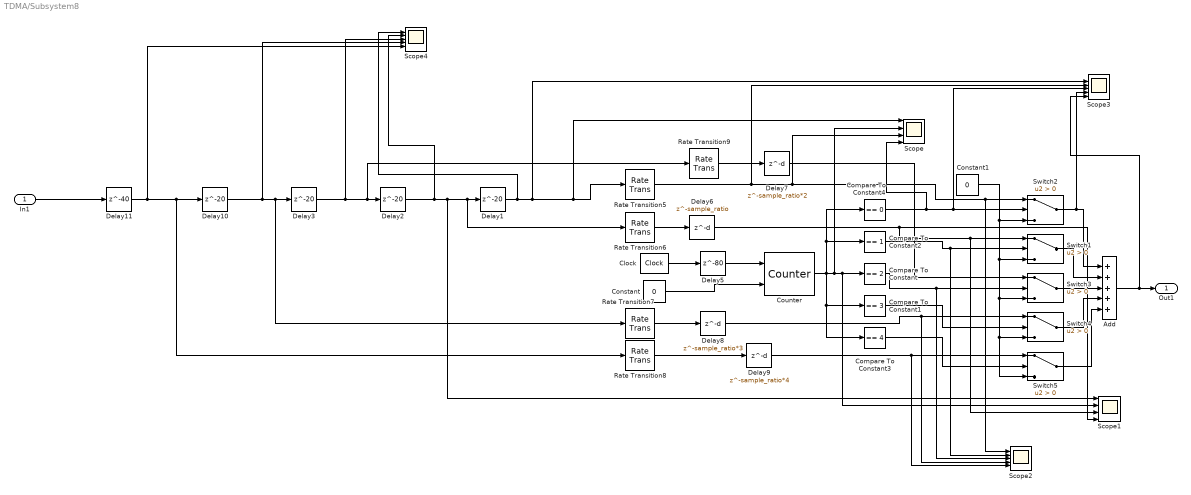
== system TDMA/Subsystem8 ==
  In1 : Inport
  Add : Sum  Inputs=+++++
  Clock : simulink_extras/Flip Flops/Clock  period=5*4/(sampling_freq)
  Compare To Constant : simulink/Logic and Bit Operations/Compare To Constant  relop===  const=2  OutDataTypeStr=boolean
  Compare To Constant1 : simulink/Logic and Bit Operations/Compare To Constant  relop===  const=3  OutDataTypeStr=boolean
  Compare To Constant2 : simulink/Logic and Bit Operations/Compare To Constant  relop===  const=1  OutDataTypeStr=boolean
  Compare To Constant3 : simulink/Logic and Bit Operations/Compare To Constant  relop===  const=4  OutDataTypeStr=boolean
  Compare To Constant4 : simulink/Logic and Bit Operations/Compare To Constant  relop===  const=0  OutDataTypeStr=boolean
  Constant : Constant  Value=0
  Constant1 : Constant  Value=0  SampleTime=25e-9
  Counter : dspswit3/Counter  Direction=Up  CountEvent=Rising edge  CounterSize=User defined  MaxCount=4  InitialCount=0  Output=Count  HitValue=32  ResetInput=on  SamplesPerFrame=1  Ts=1  CntDtype=double  HitDtype=Logical
  Delay{1..3,10} (4 alike) : Delay  DelayLength=20  SampleTime=1/(sampling_freq*5)
  Delay11 : Delay  DelayLength=40  SampleTime=1/(sampling_freq*5)
  Delay5 : Delay  DelayLength=80  SampleTime=1/(sampling_freq)
  Delay6 : Delay  DelayLength=sample_ratio  SampleTime=1/(sampling_freq)
  Delay7 : Delay  DelayLength=sample_ratio*2  SampleTime=1/(sampling_freq)
  Delay8 : Delay  DelayLength=sample_ratio*3  SampleTime=1/(sampling_freq)
  Delay9 : Delay  DelayLength=sample_ratio*4  SampleTime=1/(sampling_freq)
  Rate Transition{5..9} (5 alike) : RateTransition  OutPortSampleTime=1/(data_rate)
  Scope : Scope  NumInputPorts=4
  Scope1 : Scope  NumInputPorts=4
  Scope2 : Scope  NumInputPorts=5
  Scope3 : Scope  NumInputPorts=6
  Scope4 : Scope  NumInputPorts=5
  Switch{1..5} (5 alike) : Switch  Criteria=u2 > Threshold  OutDataTypeStr=fixdt(1,32,29)  RndMeth=Nearest
  Out1 : Outport
  wires:
  Switch2/1 -> Scope3/5, Add/1
  Counter/1 -> Scope/2, Scope1/2, Compare To Constant/1, Compare To Constant3/1, Compare To Constant1/1, Compare To Constant4/1, Compare To Constant2/1
  Add/1 -> Scope3/6, Out1/1
  Constant/1 -> Counter/2
  Switch3/1 -> Add/3
  Constant1/1 -> Switch4/3, Switch5/3, Switch3/3, Switch1/3, Switch2/3
  Switch5/1 -> Add/5
  Switch4/1 -> Add/4
  Compare To Constant2/1 -> Scope2/2, Switch1/2
  Compare To Constant3/1 -> Switch5/2
  Compare To Constant/1 -> Scope2/3, Switch3/2
  Switch1/1 -> Add/2
  Compare To Constant1/1 -> Switch4/2
  Compare To Constant4/1 -> Scope/4, Scope3/4, Switch2/2
  Delay1/1 -> Scope4/1, Scope3/2, Scope/1, Rate Transition5/1
  Rate Transition6/1 -> Delay6/1
  Rate Transition7/1 -> Delay8/1
  Rate Transition8/1 -> Delay9/1
  Rate Transition9/1 -> Delay7/1
  Clock/1 -> Delay5/1
  Delay5/1 -> Counter/1
  Delay2/1 -> Scope4/2, Scope1/1, Rate Transition6/1, Delay1/1
  Delay3/1 -> Scope4/3, Rate Transition9/1, Delay2/1
  Delay10/1 -> Scope4/4, Rate Transition7/1, Delay3/1
  Delay6/1 -> Scope1/4, Scope1/3, Switch1/1
  Delay7/1 -> Switch3/1
  Delay8/1 -> Scope2/4, Switch4/1
  Delay9/1 -> Scope2/5, Switch5/1
  Rate Transition5/1 -> Scope3/3, Scope2/1, Switch2/1, Scope/3
  In1/1 -> Delay11/1
  Delay11/1 -> Scope4/5, Rate Transition8/1, Delay10/1

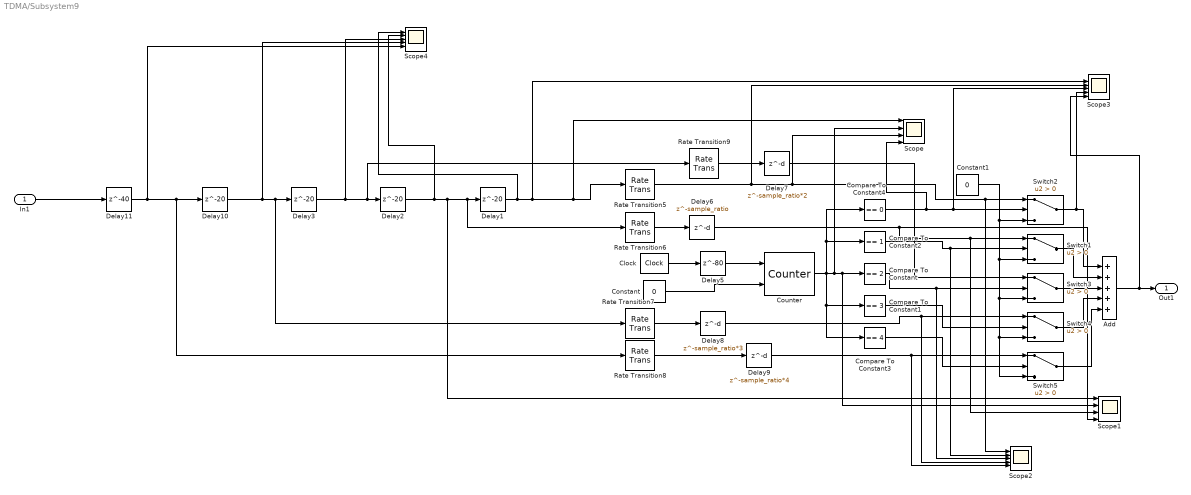
== system TDMA/Subsystem9 ==
  In1 : Inport
  Add : Sum  Inputs=+++++
  Clock : simulink_extras/Flip Flops/Clock  period=5*4/(sampling_freq)
  Compare To Constant : simulink/Logic and Bit Operations/Compare To Constant  relop===  const=2  OutDataTypeStr=boolean
  Compare To Constant1 : simulink/Logic and Bit Operations/Compare To Constant  relop===  const=3  OutDataTypeStr=boolean
  Compare To Constant2 : simulink/Logic and Bit Operations/Compare To Constant  relop===  const=1  OutDataTypeStr=boolean
  Compare To Constant3 : simulink/Logic and Bit Operations/Compare To Constant  relop===  const=4  OutDataTypeStr=boolean
  Compare To Constant4 : simulink/Logic and Bit Operations/Compare To Constant  relop===  const=0  OutDataTypeStr=boolean
  Constant : Constant  Value=0
  Constant1 : Constant  Value=0  SampleTime=25e-9
  Counter : dspswit3/Counter  Direction=Up  CountEvent=Rising edge  CounterSize=User defined  MaxCount=4  InitialCount=0  Output=Count  HitValue=32  ResetInput=on  SamplesPerFrame=1  Ts=1  CntDtype=double  HitDtype=Logical
  Delay{1..3,10} (4 alike) : Delay  DelayLength=20  SampleTime=1/(sampling_freq*5)
  Delay11 : Delay  DelayLength=40  SampleTime=1/(sampling_freq*5)
  Delay5 : Delay  DelayLength=80  SampleTime=1/(sampling_freq)
  Delay6 : Delay  DelayLength=sample_ratio  SampleTime=1/(sampling_freq)
  Delay7 : Delay  DelayLength=sample_ratio*2  SampleTime=1/(sampling_freq)
  Delay8 : Delay  DelayLength=sample_ratio*3  SampleTime=1/(sampling_freq)
  Delay9 : Delay  DelayLength=sample_ratio*4  SampleTime=1/(sampling_freq)
  Rate Transition{5..9} (5 alike) : RateTransition  OutPortSampleTime=1/(data_rate)
  Scope : Scope  NumInputPorts=4
  Scope1 : Scope  NumInputPorts=4
  Scope2 : Scope  NumInputPorts=5
  Scope3 : Scope  NumInputPorts=6
  Scope4 : Scope  NumInputPorts=5
  Switch{1..5} (5 alike) : Switch  Criteria=u2 > Threshold  OutDataTypeStr=fixdt(1,32,29)  RndMeth=Nearest
  Out1 : Outport
  wires:
  Switch2/1 -> Scope3/5, Add/1
  Counter/1 -> Scope/2, Scope1/2, Compare To Constant/1, Compare To Constant3/1, Compare To Constant1/1, Compare To Constant4/1, Compare To Constant2/1
  Add/1 -> Scope3/6, Out1/1
  Constant/1 -> Counter/2
  Switch3/1 -> Add/3
  Constant1/1 -> Switch4/3, Switch5/3, Switch3/3, Switch1/3, Switch2/3
  Switch5/1 -> Add/5
  Switch4/1 -> Add/4
  Compare To Constant2/1 -> Scope2/2, Switch1/2
  Compare To Constant3/1 -> Switch5/2
  Compare To Constant/1 -> Scope2/3, Switch3/2
  Switch1/1 -> Add/2
  Compare To Constant1/1 -> Switch4/2
  Compare To Constant4/1 -> Scope/4, Scope3/4, Switch2/2
  Delay1/1 -> Scope4/1, Scope3/2, Scope/1, Rate Transition5/1
  Rate Transition6/1 -> Delay6/1
  Rate Transition7/1 -> Delay8/1
  Rate Transition8/1 -> Delay9/1
  Rate Transition9/1 -> Delay7/1
  Clock/1 -> Delay5/1
  Delay5/1 -> Counter/1
  Delay2/1 -> Scope4/2, Scope1/1, Rate Transition6/1, Delay1/1
  Delay3/1 -> Scope4/3, Rate Transition9/1, Delay2/1
  Delay10/1 -> Scope4/4, Rate Transition7/1, Delay3/1
  Delay6/1 -> Scope1/4, Scope1/3, Switch1/1
  Delay7/1 -> Switch3/1
  Delay8/1 -> Scope2/4, Switch4/1
  Delay9/1 -> Scope2/5, Switch5/1
  Rate Transition5/1 -> Scope3/3, Scope2/1, Switch2/1, Scope/3
  In1/1 -> Delay11/1
  Delay11/1 -> Scope4/5, Rate Transition8/1, Delay10/1

== system TDMA/Carrier Signal/NCO ==
  Add : Sum  AccumDataTypeStr=double
  Constant : Constant  Value=nco_t  OutDataTypeStr=double  SampleTime=1/(sampling_freq*5)
  Data Type Conversion : DataTypeConversion  OutMin=[0]  OutMax=[2]  OutDataTypeStr=fixdt(0,8)
  Delay1 : Delay  DelayLength=1  InitialCondition=0  UseCircularBuffer=on  SampleTime=1/(sampling_freq*5)
  Delay2 : Delay  DelayLength=1  InitialCondition=0  UseCircularBuffer=on  SampleTime=1/(sampling_freq*5)
  Sine Lookup : simulink/Lookup Tables/Sine  Formula=sin(2*pi*u) and cos(2*pi*u)  NumDataPoints=(2^3)+1  OutputWordLength=8  InternalRulePriority=Speed
  Out2 : Outport
  Out1 : Outport  Port=2
  wires:
  Delay1/1 -> Add/2
  Constant/1 -> Add/1
  Add/1 -> Delay1/1, Data Type Conversion/1
  Data Type Conversion/1 -> Delay2/1
  Sine Lookup/2 -> Out2/1
  Sine Lookup/1 -> Out1/1
  Delay2/1 -> Sine Lookup/1

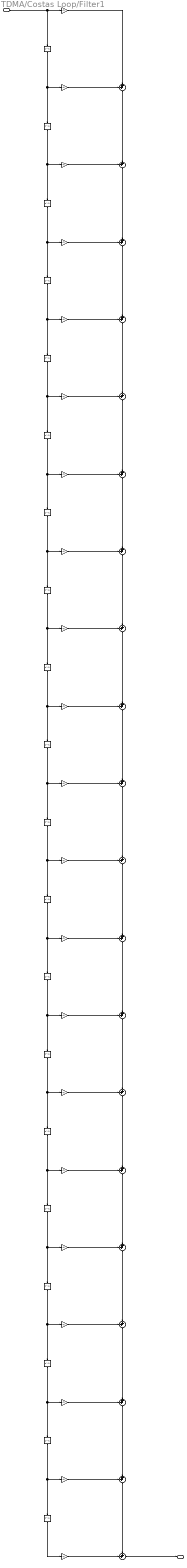
== system TDMA/Costas Loop/Filter1 ==
  Input : Inport
  BodyDelay{2..21} (20 alike) : Delay  DelayLength=1  InitialCondition=0  InputProcessing=Columns as channels (frame based)
  BodyLSum{2..21} (20 alike) : Sum  Inputs=++|  RndMeth=Nearest  SaturateOnIntegerOverflow=on  OutDataTypeStr=Inherit: Same as first input
  b(1) : Gain  Gain=coeff_t(1)  ParamDataTypeStr=double  RndMeth=Nearest  SaturateOnIntegerOverflow=on  OutDataTypeStr=Inherit: Same as input
  b(10) : Gain  Gain=coeff_t(10)  ParamDataTypeStr=double  RndMeth=Nearest  SaturateOnIntegerOverflow=on  OutDataTypeStr=Inherit: Same as input
  b(11) : Gain  Gain=coeff_t(11)  ParamDataTypeStr=double  RndMeth=Nearest  SaturateOnIntegerOverflow=on  OutDataTypeStr=Inherit: Same as input
  b(12) : Gain  Gain=coeff_t(12)  ParamDataTypeStr=double  RndMeth=Nearest  SaturateOnIntegerOverflow=on  OutDataTypeStr=Inherit: Same as input
  b(13) : Gain  Gain=coeff_t(13)  ParamDataTypeStr=double  RndMeth=Nearest  SaturateOnIntegerOverflow=on  OutDataTypeStr=Inherit: Same as input
  b(14) : Gain  Gain=coeff_t(14)  ParamDataTypeStr=double  RndMeth=Nearest  SaturateOnIntegerOverflow=on  OutDataTypeStr=Inherit: Same as input
  b(15) : Gain  Gain=coeff_t(15)  ParamDataTypeStr=double  RndMeth=Nearest  SaturateOnIntegerOverflow=on  OutDataTypeStr=Inherit: Same as input
  b(16) : Gain  Gain=coeff_t(16)  ParamDataTypeStr=double  RndMeth=Nearest  SaturateOnIntegerOverflow=on  OutDataTypeStr=Inherit: Same as input
  b(17) : Gain  Gain=coeff_t(17)  ParamDataTypeStr=double  RndMeth=Nearest  SaturateOnIntegerOverflow=on  OutDataTypeStr=Inherit: Same as input
  b(18) : Gain  Gain=coeff_t(18)  ParamDataTypeStr=double  RndMeth=Nearest  SaturateOnIntegerOverflow=on  OutDataTypeStr=Inherit: Same as input
  b(19) : Gain  Gain=coeff_t(19)  ParamDataTypeStr=double  RndMeth=Nearest  SaturateOnIntegerOverflow=on  OutDataTypeStr=Inherit: Same as input
  b(2) : Gain  Gain=coeff_t(2)  ParamDataTypeStr=double  RndMeth=Nearest  SaturateOnIntegerOverflow=on  OutDataTypeStr=Inherit: Same as input
  b(20) : Gain  Gain=coeff_t(20)  ParamDataTypeStr=double  RndMeth=Nearest  SaturateOnIntegerOverflow=on  OutDataTypeStr=Inherit: Same as input
  b(21) : Gain  Gain=coeff_t(21)  ParamDataTypeStr=double  RndMeth=Nearest  SaturateOnIntegerOverflow=on  OutDataTypeStr=Inherit: Same as input
  b(3) : Gain  Gain=coeff_t(3)  ParamDataTypeStr=double  RndMeth=Nearest  SaturateOnIntegerOverflow=on  OutDataTypeStr=Inherit: Same as input
  b(4) : Gain  Gain=coeff_t(4)  ParamDataTypeStr=double  RndMeth=Nearest  SaturateOnIntegerOverflow=on  OutDataTypeStr=Inherit: Same as input
  b(5) : Gain  Gain=coeff_t(5)  ParamDataTypeStr=double  RndMeth=Nearest  SaturateOnIntegerOverflow=on  OutDataTypeStr=Inherit: Same as input
  b(6) : Gain  Gain=coeff_t(6)  ParamDataTypeStr=double  RndMeth=Nearest  SaturateOnIntegerOverflow=on  OutDataTypeStr=Inherit: Same as input
  b(7) : Gain  Gain=coeff_t(7)  ParamDataTypeStr=double  RndMeth=Nearest  SaturateOnIntegerOverflow=on  OutDataTypeStr=Inherit: Same as input
  b(8) : Gain  Gain=coeff_t(8)  ParamDataTypeStr=double  RndMeth=Nearest  SaturateOnIntegerOverflow=on  OutDataTypeStr=Inherit: Same as input
  b(9) : Gain  Gain=coeff_t(9)  ParamDataTypeStr=double  RndMeth=Nearest  SaturateOnIntegerOverflow=on  OutDataTypeStr=Inherit: Same as input
  Output : Outport
  wires:
  Input/1 -> b(1)/1, BodyDelay2/1
  b(1)/1 -> BodyLSum2/2
  BodyDelay2/1 -> b(2)/1, BodyDelay3/1
  b(2)/1 -> BodyLSum2/1
  BodyLSum2/1 -> BodyLSum3/2
  BodyDelay3/1 -> b(3)/1, BodyDelay4/1
  b(3)/1 -> BodyLSum3/1
  BodyLSum3/1 -> BodyLSum4/2
  BodyDelay4/1 -> b(4)/1, BodyDelay5/1
  b(4)/1 -> BodyLSum4/1
  BodyLSum4/1 -> BodyLSum5/2
  BodyDelay5/1 -> b(5)/1, BodyDelay6/1
  b(5)/1 -> BodyLSum5/1
  BodyLSum5/1 -> BodyLSum6/2
  BodyDelay6/1 -> b(6)/1, BodyDelay7/1
  b(6)/1 -> BodyLSum6/1
  BodyLSum6/1 -> BodyLSum7/2
  BodyDelay7/1 -> b(7)/1, BodyDelay8/1
  b(7)/1 -> BodyLSum7/1
  BodyLSum7/1 -> BodyLSum8/2
  BodyDelay8/1 -> b(8)/1, BodyDelay9/1
  b(8)/1 -> BodyLSum8/1
  BodyLSum8/1 -> BodyLSum9/2
  BodyDelay9/1 -> b(9)/1, BodyDelay10/1
  b(9)/1 -> BodyLSum9/1
  BodyLSum9/1 -> BodyLSum10/2
  BodyDelay10/1 -> b(10)/1, BodyDelay11/1
  b(10)/1 -> BodyLSum10/1
  BodyLSum10/1 -> BodyLSum11/2
  BodyDelay11/1 -> b(11)/1, BodyDelay12/1
  b(11)/1 -> BodyLSum11/1
  BodyLSum11/1 -> BodyLSum12/2
  BodyDelay12/1 -> b(12)/1, BodyDelay13/1
  b(12)/1 -> BodyLSum12/1
  BodyLSum12/1 -> BodyLSum13/2
  BodyDelay13/1 -> b(13)/1, BodyDelay14/1
  b(13)/1 -> BodyLSum13/1
  BodyLSum13/1 -> BodyLSum14/2
  BodyDelay14/1 -> b(14)/1, BodyDelay15/1
  b(14)/1 -> BodyLSum14/1
  BodyLSum14/1 -> BodyLSum15/2
  BodyDelay15/1 -> b(15)/1, BodyDelay16/1
  b(15)/1 -> BodyLSum15/1
  BodyLSum15/1 -> BodyLSum16/2
  BodyDelay16/1 -> b(16)/1, BodyDelay17/1
  b(16)/1 -> BodyLSum16/1
  BodyLSum16/1 -> BodyLSum17/2
  BodyDelay17/1 -> b(17)/1, BodyDelay18/1
  b(17)/1 -> BodyLSum17/1
  BodyLSum17/1 -> BodyLSum18/2
  BodyDelay18/1 -> b(18)/1, BodyDelay19/1
  b(18)/1 -> BodyLSum18/1
  BodyLSum18/1 -> BodyLSum19/2
  BodyDelay19/1 -> b(19)/1, BodyDelay20/1
  b(19)/1 -> BodyLSum19/1
  BodyLSum19/1 -> BodyLSum20/2
  BodyDelay20/1 -> b(20)/1, BodyDelay21/1
  b(20)/1 -> BodyLSum20/1
  BodyLSum20/1 -> BodyLSum21/1
  BodyDelay21/1 -> b(21)/1
  b(21)/1 -> BodyLSum21/2
  BodyLSum21/1 -> Output/1
